simulink model "aaa1"  (R2021b)
settings: Solver=VariableStepAuto  StartTime=0.0  StopTime=180  RelTol=1e-3
settings Model: Creator=郭义月  LastModifiedBy=郭义月

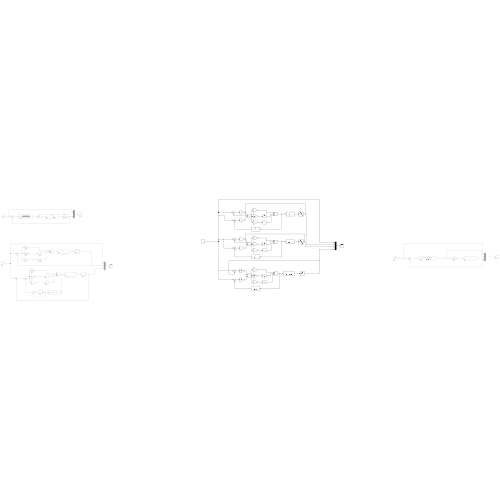
[thumbnail: Simulink's stored preview of the top-level diagram]
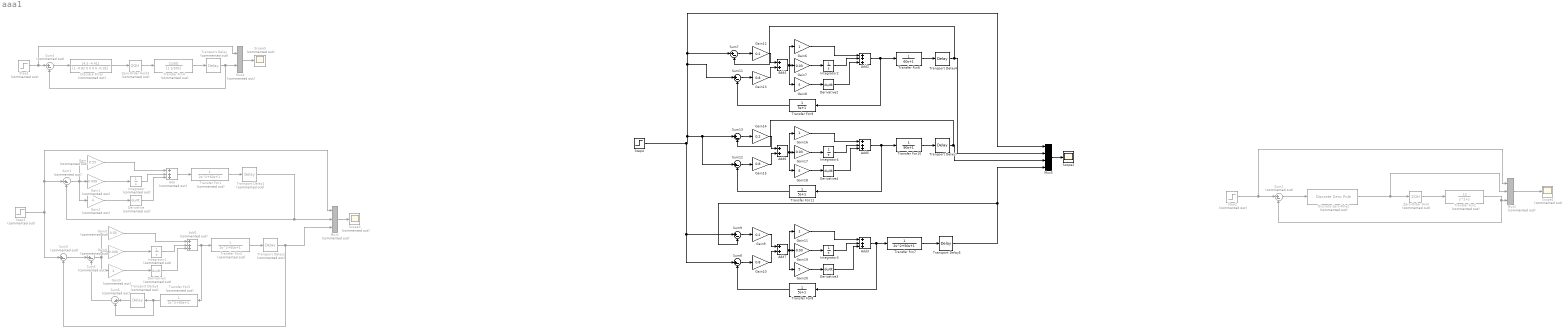
== system aaa1 ==
  Add : Sum  Commented=on  Inputs=+++
  Add1 : Sum  Commented=on  Inputs=+++
  Add2 : Sum  Inputs=+++
  Add3 : Sum  Inputs=+++
  Add4 : Sum
  Add5 : Sum  Inputs=+++
  Add6 : Sum
  Add7 : Sum
  Derivative : Derivative  Commented=on
  Derivative1 : Derivative  Commented=on
  Derivative2 : Derivative
  Derivative3 : Derivative
  Derivative4 : Derivative
  Discrete Zero-Pole2 : DiscreteZeroPole  Commented=on  Zeros=[0.3679]  Poles=[-0.718]  Gain=0.7  SampleTime=-1
  Discrete Filter : DiscreteFilter  Commented=on  Numerator=[4.5 -4.41]  Denominator=[1 -0.82 0 0 0 0 -0.18]
  Gain : Gain  Commented=on  Gain=0.55
  Gain1 : Gain  Commented=on  Gain=0.008
  Gain10 : Gain  Gain=0.8
  Gain11 : Gain
  Gain12 : Gain  Gain=0.2
  Gain13 : Gain  Gain=0.8
  Gain14 : Gain  Gain=0.2
  Gain15 : Gain  Gain=0.8
  Gain16 : Gain
  Gain17 : Gain  Gain=0.03
  Gain18 : Gain  Gain=5
  Gain19 : Gain  Gain=0.03
  Gain2 : Gain  Commented=on  Gain=4
  Gain20 : Gain  Gain=5
  Gain3 : Gain  Commented=on  Gain=0.55
  Gain4 : Gain  Commented=on  Gain=0.008
  Gain5 : Gain  Commented=on  Gain=4
  Gain6 : Gain
  Gain7 : Gain  Gain=0.03
  Gain8 : Gain  Gain=5
  Gain9 : Gain  Gain=0.2
  Integrator : Integrator  Commented=on
  Integrator1 : Integrator  Commented=on
  Integrator2 : Integrator
  Integrator3 : Integrator
  Integrator4 : Integrator
  Mux1 : Mux  Commented=on  Inputs=3
  Mux2 : Mux  Commented=on  Inputs=3
  Mux3 : Mux
  Mux4 : Mux  Commented=on  Inputs=2
  Scope1 : Scope  Commented=on
  Scope2 : Scope
  Scope3 : Scope  Commented=on
  Scope5 : Scope  Commented=on
  Step1 : Step  Commented=on  SampleTime=0
  Step2 : Step  Commented=on  SampleTime=0
  Step3 : Step  Commented=on  SampleTime=0
  Step4 : Step  SampleTime=0
  Sum{1..6} (6 alike) : Sum  Commented=on  Inputs=|+-
  Sum{7..9,11..13} (6 alike) : Sum  Inputs=|+-
  Transfer Fcn1 : TransferFcn  Commented=on  Denominator=[2 60 1]
  Transfer Fcn10 : TransferFcn  Denominator=[90 1]
  Transfer Fcn11 : TransferFcn  Denominator=[5 1]
  Transfer Fcn2 : TransferFcn  Commented=on  Numerator=[10]  Denominator=[1 1 0]
  Transfer Fcn3 : TransferFcn  Commented=on  Denominator=[2 60 1]
  Transfer Fcn4 : TransferFcn  Commented=on  Numerator=[1/50]  Denominator=[1 1/100]
  Transfer Fcn5 : TransferFcn  Commented=on  Denominator=[2 60 1]
  Transfer Fcn6 : TransferFcn  Denominator=[60 1]
  Transfer Fcn7 : TransferFcn  Denominator=[2 50 1]
  Transfer Fcn8 : TransferFcn  Denominator=[5 1]
  Transfer Fcn9 : TransferFcn  Denominator=[5 1]
  Transport Delay : TransportDelay  Commented=on  DelayTime=10
  Transport Delay1 : TransportDelay  Commented=on  DelayTime=30
  Transport Delay2 : TransportDelay  Commented=on  DelayTime=30
  Transport Delay3 : TransportDelay  Commented=on  DelayTime=30
  Transport Delay4 : TransportDelay  DelayTime=30
  Transport Delay5 : TransportDelay  DelayTime=30
  Transport Delay7 : TransportDelay  DelayTime=30
  Zero-Order Hold : ZeroOrderHold  Commented=on  SampleTime=-1
  Zero-Order Hold3 : ZeroOrderHold  Commented=on  SampleTime=-1
  wires:
  Zero-Order Hold/1 -> Transfer Fcn2/1
  Transfer Fcn2/1 -> Mux2/3, Sum2/2
  Step2/1 -> Mux2/1, Sum2/1
  Mux2/1 -> Scope1/1
  Discrete Zero-Pole2/1 -> Mux2/2, Zero-Order Hold/1
  Sum2/1 -> Discrete Zero-Pole2/1
  Discrete Filter/1 -> Zero-Order Hold3/1
  Mux4/1 -> Scope5/1
  Step1/1 -> Mux4/1, Sum4/1
  Sum4/1 -> Discrete Filter/1
  Zero-Order Hold3/1 -> Transfer Fcn4/1
  Transfer Fcn4/1 -> Transport Delay/1
  Transport Delay/1 -> Sum4/2, Mux4/2
  Mux1/1 -> Scope3/1
  Gain1/1 -> Integrator/1
  Gain2/1 -> Derivative/1
  Derivative/1 -> Add/3
  Integrator/1 -> Add/2
  Gain/1 -> Add/1
  Sum1/1 -> Gain2/1, Gain1/1, Gain/1
  Add/1 -> Transfer Fcn1/1
  Transfer Fcn1/1 -> Transport Delay1/1
  Step3/1 -> Sum3/1, Sum1/1, Mux1/1
  Sum3/1 -> Sum5/1
  Sum5/1 -> Gain4/1, Gain3/1, Gain5/1
  Gain4/1 -> Integrator1/1
  Gain5/1 -> Derivative1/1
  Gain3/1 -> Add1/1
  Integrator1/1 -> Add1/2
  Derivative1/1 -> Add1/3
  Add1/1 -> Transfer Fcn5/1, Transfer Fcn3/1
  Transfer Fcn3/1 -> Transport Delay2/1
  Transport Delay1/1 -> Sum1/2, Mux1/2
  Transfer Fcn5/1 -> Sum6/2, Transport Delay3/1
  Transport Delay3/1 -> Sum6/1
  Sum6/1 -> Sum5/2
  Transport Delay2/1 -> Mux1/3, Sum3/2
  Mux3/1 -> Scope2/1
  Add4/1 -> Gain8/1, Gain6/1, Gain7/1
  Gain12/1 -> Add4/1
  Gain13/1 -> Add4/2
  Sum11/1 -> Gain13/1
  Gain7/1 -> Integrator2/1
  Gain8/1 -> Derivative2/1
  Gain6/1 -> Add2/1
  Integrator2/1 -> Add2/2
  Derivative2/1 -> Add2/3
  Add2/1 -> Transfer Fcn9/1, Transfer Fcn6/1
  Transfer Fcn6/1 -> Transport Delay4/1
  Transfer Fcn9/1 -> Sum11/2
  Sum7/1 -> Gain12/1
  Step4/1 -> Sum9/1, Sum8/1, Sum12/1, Sum13/1, Sum11/1, Sum7/1, Mux3/1
  Transport Delay4/1 -> Sum7/2, Mux3/2
  Sum13/1 -> Gain14/1
  Sum12/1 -> Gain15/1
  Add6/1 -> Gain18/1, Gain16/1, Gain17/1
  Gain14/1 -> Add6/1
  Gain15/1 -> Add6/2
  Gain17/1 -> Integrator4/1
  Gain18/1 -> Derivative4/1
  Gain16/1 -> Add5/1
  Integrator4/1 -> Add5/2
  Derivative4/1 -> Add5/3
  Add5/1 -> Transfer Fcn11/1, Transfer Fcn10/1
  Transfer Fcn10/1 -> Transport Delay7/1
  Transport Delay7/1 -> Sum13/2, Mux3/3
  Transport Delay5/1 -> Sum9/2, Mux3/4
  Sum9/1 -> Gain9/1
  Sum8/1 -> Gain10/1
  Add7/1 -> Gain20/1, Gain11/1, Gain19/1
  Gain9/1 -> Add7/1
  Gain10/1 -> Add7/2
  Gain19/1 -> Integrator3/1
  Gain11/1 -> Add3/1
  Integrator3/1 -> Add3/2
  Derivative3/1 -> Add3/3
  Gain20/1 -> Derivative3/1
  Add3/1 -> Transfer Fcn8/1, Transfer Fcn7/1
  Transfer Fcn7/1 -> Transport Delay5/1
  Transfer Fcn11/1 -> Sum12/2
  Transfer Fcn8/1 -> Sum8/2
